simulink model "rail_ver01"  (R2018a)
settings: Solver=VariableStepAuto  StartTime=0.0  StopTime=inf  RelTol=1e-3
InitFcn:
  | %run('settingParams_ver04.m')
StopFcn:
  | run('AutomoveData.m')
values from neighbouring files (symbols this model uses):
  acceleration = 100    [settingParams_demo.m]
  armInitPos = [120,0,280,0,0,0,10,20]    [settingParams_demo.m]
  correct = [15, -50, 110, 35, 90, 90]    [settingParams_demo.m]
  direction = -1    [settingParams_demo.m]
  dt = 0.1    [settingParams_demo.m]
  dummyDepth = 600    [settingParams_demo.m]
  erosion = 1    [settingParams_demo.m]
  first = 0    [settingParams_demo.m]
  limit_range_ANA = [h2_1, h2_2, w2_r1, w2_r2, w2_l1, w2_l2]    [settingParams_demo.m]
  limit_range_IMG = [h1_1, h1_2, w1_r1, w1_r2, w1_l1, w1_l2]    [settingParams_demo.m]
  pitchAdd = [0,0,50,0,60,0]    [settingParams_demo.m]
  range_m = range / 1000    (= 0.9)    [settingParams_demo.m]
  range_mm = range    (= 900)    [settingParams_demo.m]
  relationOfArmCam = [530, 330, -100]    [settingParams_demo.m]
  termDistance = railDistance - robotLength - first    (= 0.8)    [settingParams_demo.m]
  translationVector = [0, 0, 0]    [settingParams_demo.m]
  value = [HMin, HMax, SMin, SMax, VMin, VMax]    [settingParams_demo.m]
  velocity = 50    [settingParams_demo.m]
undefined symbols (not defined in the file or in its folder): BodyIndexFrame, BodyTrackingID, ColorJointIndices, DepthJointIndices, gray, HandLeftConfidence, HandLeftState, HandRightConfidence, HandRightState, IsBodyTracked, JointPositions, JointTrackingState, none, serial, strel, videoinput
libraries: instrumentlib x6, simulink x4, visiontextngfix x3, visionmorphops x2, imaqlib x2, visionstatistics x1, sldrtlib x1
(part 1 of 2)
settings Model: Creator=tomato  LastModifiedBy=tomatoPC
settings CodeAppCC: StateflowObjectComments=on

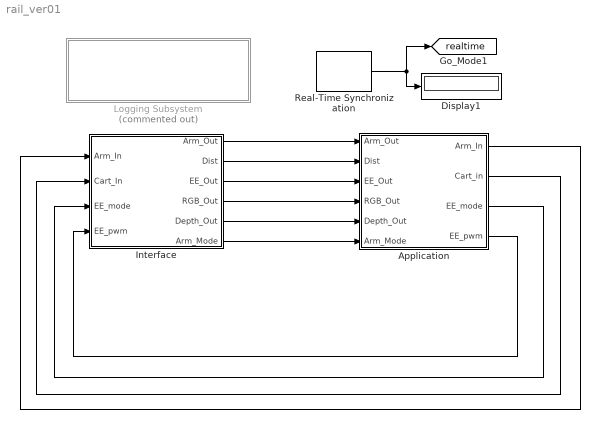
== system rail_ver01 ==
  Application : Subsystem
  Display1 : Display
  Interface : Subsystem
  Logging Subsystem : Subsystem  Commented=on
  Real-Time Synchronization : sldrtlib/Real-Time Synchronization  SampleTime=dt  MaxMissedTicks=inf  ShowMissedTicks=on  YieldWhenWaiting=off
  tag scope: realtime=global
  wires:
  Real-Time Synchronization/1 -> [realtime], Display1/1
  Application/1(Arm_In) -> Interface/1(Arm_In)
  Application/3(EE_mode) -> Interface/3(EE_mode)
  Application/2(Cart_in) -> Interface/2(Cart_In)
  Interface/1(Arm_Out) -> Application/1(Arm_Out)
  Interface/2(Dist) -> Application/2(Dist)
  Interface/3(EE_Out) -> Application/3(EE_Out)
  Interface/4(RGB_Out) -> Application/4(RGB_Out)
  Interface/5(Depth_Out) -> Application/5(Depth_Out)
  Interface/6(Arm_Mode) -> Application/6(Arm_Mode)
  Application/4(EE_pwm) -> Interface/4(EE_pwm)

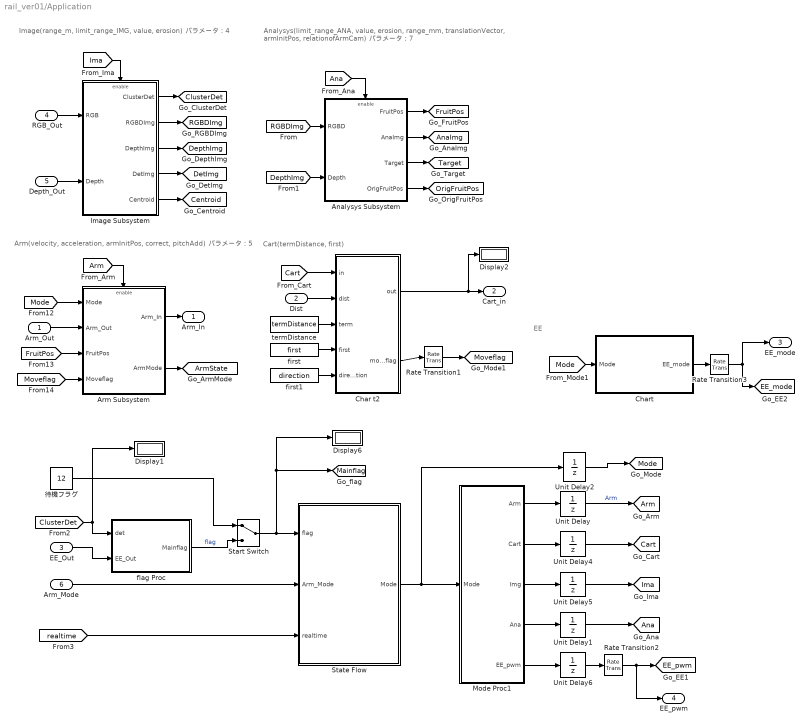
== system rail_ver01/Application ==
  note: Cart(termDistance, first)
  note: Image(range_m, limit_range_IMG, value, erosion)
      | パラメータ：4
  note: Analysys(limit_range_ANA, value, erosion, range_mm,
      |              translationVector, armInitPos, relationofArmCam)
      | パラメータ：7
  note: Arm(velocity, acceleration, armInitPos, correct, pitchAdd)
      | パラメータ：5
  note: EE
  Arm_Out : Inport
  Dist : Inport  Port=2
  EE_Out : Inport  Port=3
  RGB_Out : Inport  Port=4
  Depth_Out : Inport  Port=5
  Arm_Mode : Inport  Port=6
  Analysys Subsystem : Subsystem  TreatAsAtomicUnit=on
  Arm Subsystem : Subsystem  TreatAsAtomicUnit=on
  Char t2 : Stateflow chart  TreatAsAtomicUnit=on
  Chart : Stateflow chart  TreatAsAtomicUnit=on
  Display1 : Display
  Display2 : Display
  Display6 : Display
  Image Subsystem : Subsystem  TreatAsAtomicUnit=on
  Mode Proc1 : MATLAB Function  TreatAsAtomicUnit=on
  Rate Transition1 : RateTransition  OutPortSampleTime=0.1
  Rate Transition2 : RateTransition  OutPortSampleTime=0.1
  Rate Transition3 : RateTransition  OutPortSampleTime=0.1
  Start Switch : ManualSwitch
  State Flow : Stateflow chart  TreatAsAtomicUnit=on
  Unit Delay{,1..2,4..6} (6 alike) : UnitDelay  SampleTime=-1
  first : Constant  Value=first  SampleTime=dt
  first1 : Constant  Value=direction  SampleTime=dt
  flag Proc : MATLAB Function  TreatAsAtomicUnit=on
  termDistance : Constant  Value=termDistance  SampleTime=dt
  待機フラグ : Constant  Value=12
  Arm_In : Outport
  Cart_in : Outport  Port=2
  EE_mode : Outport  Port=3
  EE_pwm : Outport  Port=4
  tag scope: Ana=global, AnaImg=global, Arm=global, ArmState=global, Cart=global, Centroid=global, ClusterDet=global, DepthImg=global, DetImg=global, EE_mode=global, EE_pwm=global, FruitPos=global, Ima=global, Mainflag=global, Mode=global, Moveflag=global, OrigFruitPos=global, RGBDImg=global, Target=global
  wires:
  Mode Proc1/1(Arm) -> Unit Delay/1
  Mode Proc1/2(Cart) -> Unit Delay4/1
  Mode Proc1/3(Img) -> Unit Delay5/1
  Mode Proc1/5(EE_pwm) -> Unit Delay6/1
  Unit Delay/1 -> [Arm]  "Arm"
  Unit Delay5/1 -> [Ima]
  flag Proc/1(Mainflag) -> Start Switch/2  "flag"
  Start Switch/1 -> [Mainflag], Display6/1, State Flow/1(flag)
  待機フラグ/1 -> Start Switch/1
  [Arm] -> Arm Subsystem/Enable
  Arm Subsystem/1(Arm_In) -> Arm_In/1
  [FruitPos] -> Arm Subsystem/3(FruitPos)
  EE_Out/1 -> flag Proc/2(EE_Out)
  [ClusterDet] -> Display1/1, flag Proc/1(det)
  RGB_Out/1 -> Image Subsystem/1(RGB)
  Image Subsystem/1(ClusterDet) -> [ClusterDet]
  [Ima] -> Image Subsystem/Enable
  Image Subsystem/2(RGBDImg) -> [RGBDImg]
  Analysys Subsystem/1(FruitPos) -> [FruitPos]
  Mode Proc1/4(Ana) -> Unit Delay1/1
  Unit Delay1/1 -> [Ana]
  [Ana] -> Analysys Subsystem/Enable
  [RGBDImg] -> Analysys Subsystem/1(RGBD)
  Depth_Out/1 -> Image Subsystem/2(Depth)
  Arm_Mode/1 -> State Flow/2(Arm_Mode)
  State Flow/1(Mode) -> Unit Delay2/1, Mode Proc1/1(Mode)
  Unit Delay2/1 -> [Mode]
  Image Subsystem/3(DepthImg) -> [DepthImg]
  [DepthImg] -> Analysys Subsystem/2(Depth)
  Arm Subsystem/2(ArmMode) -> [ArmState]
  [Mode] -> Arm Subsystem/1(Mode)
  Arm_Out/1 -> Arm Subsystem/2(Arm_Out)
  Dist/1 -> Char t2/2(dist)
  Char t2/1(out) -> Display2/1, Cart_in/1
  termDistance/1 -> Char t2/3(term)
  first/1 -> Char t2/4(first)
  Unit Delay4/1 -> [Cart]
  [Cart] -> Char t2/1(in)
  [Moveflag] -> Arm Subsystem/4(Moveflag)
  Char t2/2(moveflag) -> Rate Transition1/1
  Image Subsystem/4(DetImg) -> [DetImg]
  Image Subsystem/5(Centroid) -> [Centroid]
  Analysys Subsystem/2(AnaImg) -> [AnaImg]
  Analysys Subsystem/3(Target) -> [Target]
  Analysys Subsystem/4(OrigFruitPos) -> [OrigFruitPos]
  [Mode] -> Chart/1(Mode)
  Chart/1(EE_mode) -> Rate Transition3/1
  Rate Transition1/1 -> [Moveflag]
  Unit Delay6/1 -> Rate Transition2/1
  Rate Transition3/1 -> [EE_mode], EE_mode/1
  Rate Transition2/1 -> EE_pwm/1, [EE_pwm]
  [realtime] -> State Flow/3(realtime)
  first1/1 -> Char t2/5(direction)

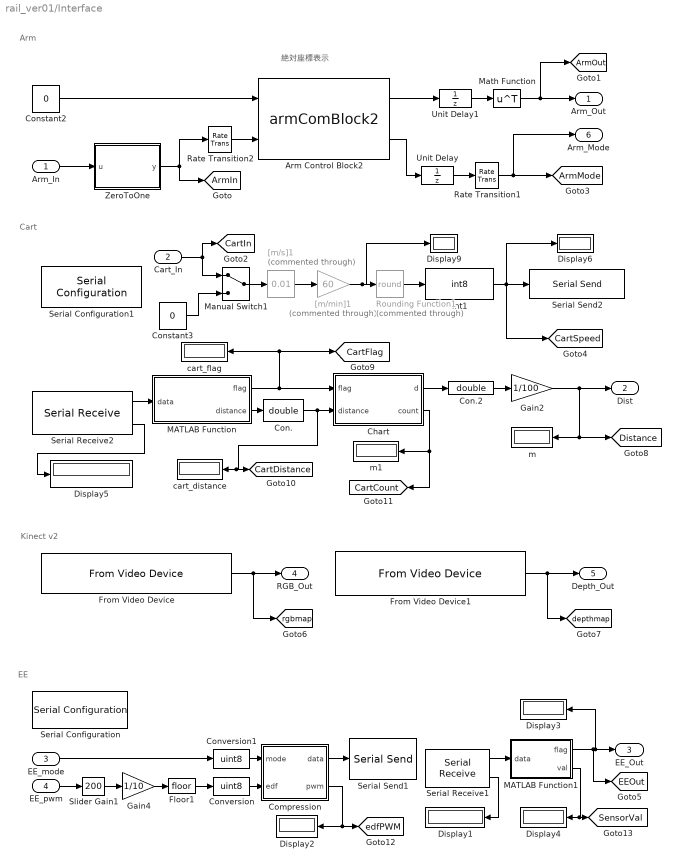
== system rail_ver01/Interface ==
  note: Kinect v2
  note: Arm
  note: 絶対座標表示
  note: EE
  note: Cart
  Arm_In : Inport
  Cart_In : Inport  Port=2
  EE_mode : Inport  Port=3
  EE_pwm : Inport  Port=4
  Arm Control Block2 : M-S-Function  FunctionName=armComBlock2  Parameters=comport, baud, tempPos  mask{comport='COM7', baud=115200, tempPos=armInitPos}
      mask prompts: comport "Port Number"; baud "Baudrate"; tempPos "Temporary Position"
      mask help: Canon Arm Control Block ver.0.8
      mask Display:
      | disp('Arm Control Block');
      | port_label('input',1,'Calib.');
      | port_label('input',2,'Target');
      | port_label('output',1,'Pos.');
      | port_label('output',2,'Moved');
  Chart : Stateflow chart  TreatAsAtomicUnit=on
  Compression : MATLAB Function  TreatAsAtomicUnit=on
  Con. : DataTypeConversion  OutDataTypeStr=double
  Con.2 : DataTypeConversion  OutDataTypeStr=double
  Constant2 : Constant  Value=0  SampleTime=0.1
  Constant3 : Constant  Value=0  SampleTime=dt
  Conversion : DataTypeConversion  OutDataTypeStr=uint8
  Conversion1 : DataTypeConversion  OutDataTypeStr=uint8
  Display{1..6,9} (7 alike) : Display
  Floor1 : Rounding
  From Video Device : imaqlib/From Video Device  DeviceMenu=kinect 1 (Kinect V2 Color Sensor)  Device=kinect 1 (Kinect V2 Color Sensor)  ObjConstructor=videoinput('kinect', 1)  VideoFormatMenu=BGR_1920x1080  VideoFormat=BGR_1920x1080  VideoSource=Kinect V2 Color Source  ROIPosition=[0 0 1080 1920]  EnableHWTrigger=off  TriggerConfiguration=kinect 1 (Kinect V2 Color Sensor)  SampleTime=0.1  OutputPortsMode=One multidimensional signal  DataType=uint8  CanDoHWTrigger=no  ReturnedColorSpace=rgb  BlockHandle=6.0001  ROIWidth=1920  ROIHeight=1080  ROIColumn=0  ROIRow=0  EngXMLPath=C:\Program Files\MATLAB\R2018a\toolbox\imaq\imaq\private  DevXMLPath=C:\ProgramData\MATLAB\SupportPackages\R2018a\toolbox\imaq\supportpackages\kinectruntime\adaptor\win64  EngLibPath=C:\Program Files\MATLAB\R2018a\toolbox\imaq\imaqblks\imaqmex\win64  ColorSpace=rgb  BayerSensorAlignment=grbg
      settings: SourceProductName=Image Acquisition Toolbox
  From Video Device1 : imaqlib/From Video Device  DeviceMenu=kinect 2 (Kinect V2 Depth Sensor)  Device=kinect 2 (Kinect V2 Depth Sensor)  ObjConstructor=videoinput('kinect', 2)  VideoFormatMenu=Depth_512x424  VideoFormat=Depth_512x424  VideoSource=Kinect V2 Depth Source  ROIPosition=[0 0 424 512]  EnableHWTrigger=off  TriggerConfiguration=none/none  SampleTime=0.1  OutputPortsMode=One multidimensional signal  DataType=uint16  CanDoHWTrigger=no  ReturnedColorSpace=grayscale  BlockHandle=6.0001  ROIWidth=512  ROIHeight=424  ROIColumn=0  ROIRow=0  EngXMLPath=C:\Program Files\MATLAB\R2018a\toolbox\imaq\imaq\private  DevXMLPath=C:\ProgramData\MATLAB\SupportPackages\R2018a\toolbox\imaq\supportpackages\kinectruntime\adaptor\win64  EngLibPath=C:\Program Files\MATLAB\R2018a\toolbox\imaq\imaqblks\imaqmex\win64  ColorSpace=grayscale  BayerSensorAlignment=grbg  AllMetadata=BodyIndexFrame;BodyTrackingID;ColorJointIndices;DepthJointIndices;HandLeftConfidence;HandLeftState;HandRightConfidence;HandRightState;IsBodyTracked;JointPositions;JointTrackingState
      settings: SourceProductName=Image Acquisition Toolbox
  Gain2 : Gain  Gain=1/100
  Gain4 : Gain  Gain=1/10
  MATLAB Function : MATLAB Function  TreatAsAtomicUnit=on
  MATLAB Function1 : MATLAB Function  TreatAsAtomicUnit=on
  Manual Switch1 : ManualSwitch
  Math Function : Math  Operator=transpose  SaturateOnIntegerOverflow=on
  Rate Transition1 : RateTransition  OutPortSampleTime=dt
  Rate Transition2 : RateTransition  OutPortSampleTime=dt
  Rounding Function1 : Rounding  Commented=through  Operator=round
  Serial Configuration : instrumentlib/Serial Configuration  Priority=-200000  ComPortMenu=<Please select a port...>  ComPort=COM3  ObjConstructor=serial('COM3');  BaudRate=115200  DataBits=8  Parity=none  StopBits=1  FlowControl=none  Timeout=10  ByteOrder=LittleEndian
  Serial Configuration1 : instrumentlib/Serial Configuration  Priority=-200000  ComPortMenu=<Please select a port...>  ComPort=COM5  ObjConstructor=serial('COM5');  BaudRate=115200  DataBits=8  Parity=none  StopBits=1  FlowControl=none  Timeout=10  ByteOrder=LittleEndian
  Serial Receive1 : instrumentlib/Serial Receive  ComPortMenu=<Please select a port...>  ComPort=COM3  ObjConstructor=serial('COM3');  Terminator=<none>  DataSize=1  DataType=uint8  EnableBlockingMode=off  ActionDataUnavailable=Output last received value  CustomValue=0  SampleTime=0.1
  Serial Receive2 : instrumentlib/Serial Receive  ComPortMenu=<Please select a port...>  ComPort=COM5  ObjConstructor=serial('COM5');  Terminator=<none>  DataSize=1  DataType=uint8  EnableBlockingMode=off  ActionDataUnavailable=Output last received value  CustomValue=0  SampleTime=0.1
  Serial Send1 : instrumentlib/Serial Send  ComPortMenu=<Please select a port...>  ComPort=COM3  ObjConstructor=serial('COM3');  Terminator=<none>  EnableBlockingMode=off
  Serial Send2 : instrumentlib/Serial Send  ComPortMenu=<Please select a port...>  ComPort=COM5  ObjConstructor=serial('COM5');  Terminator=<none>  EnableBlockingMode=on
  Slider Gain1 : simulink/Math Operations/Slider Gain  gain=200  low=0  high=250
  Unit Delay : UnitDelay  SampleTime=-1
  Unit Delay1 : UnitDelay  InitialCondition=[200 0 400 0 0 0]  SampleTime=-1
  ZeroToOne : MATLAB Function  TreatAsAtomicUnit=on
  "[m/min]1" : Gain  Commented=through  Gain=60
  "[m/s]1" : simulink/Math Operations/Slider Gain  Commented=through  gain=0.01  low=-0.23  high=0.23
  cart_distance : Display
  cart_flag : Display
  int1 : DataTypeConversion  OutDataTypeStr=int8
  m : Display
  m1 : Display
  Arm_Out : Outport
  Dist : Outport  Port=2
  EE_Out : Outport  Port=3
  RGB_Out : Outport  Port=4
  Depth_Out : Outport  Port=5
  Arm_Mode : Outport  Port=6
  tag scope: ArmIn=global, ArmMode=global, ArmOut=global, CartCount=global, CartDistance=global, CartFlag=global, CartIn=global, CartSpeed=global, Distance=global, EEOut=global, SensorVal=global, depthmap=global, edfPWM=global, rgbmap=global
  wires:
  Constant2/1 -> Arm Control Block2/1
  Arm Control Block2/1 -> Unit Delay1/1
  Math Function/1 -> [ArmOut], Arm_Out/1
  Unit Delay/1 -> Rate Transition1/1
  Arm Control Block2/2 -> Unit Delay/1
  Unit Delay1/1 -> Math Function/1
  Serial Receive1/2 -> Display1/1
  From Video Device/1 -> [rgbmap], RGB_Out/1
  From Video Device1/1 -> [depthmap], Depth_Out/1
  Manual Switch1/1 -> "[m/s]1"/1
  Cart_In/1 -> Manual Switch1/1, [CartIn]
  Rounding Function1/1 -> int1/1
  Constant3/1 -> Manual Switch1/2
  "[m/s]1"/1 -> "[m/min]1"/1
  int1/1 -> [CartSpeed], Serial Send2/1, Display6/1
  "[m/min]1"/1 -> Display9/1, Rounding Function1/1
  Serial Receive2/2 -> Display5/1
  Gain2/1 -> Dist/1, m/1, [Distance]
  Con.2/1 -> Gain2/1
  Serial Receive2/1 -> MATLAB Function/1(data)
  Chart/1(d) -> Con.2/1
  MATLAB Function/1(flag) -> cart_flag/1, [CartFlag], Chart/1(flag)
  MATLAB Function/2(distance) -> Con./1
  Chart/2(count) -> [CartCount], m1/1
  EE_pwm/1 -> Slider Gain1/1
  Gain4/1 -> Floor1/1
  Slider Gain1/1 -> Gain4/1
  Floor1/1 -> Conversion/1
  EE_mode/1 -> Conversion1/1
  Compression/1(data) -> Serial Send1/1
  Serial Receive1/1 -> MATLAB Function1/1(data)
  MATLAB Function1/2(val) -> [SensorVal], Display4/1
  Conversion/1 -> Compression/2(edf)
  Conversion1/1 -> Compression/1(mode)
  MATLAB Function1/1(flag) -> Display3/1, EE_Out/1, [EEOut]
  Con./1 -> cart_distance/1, [CartDistance], Chart/2(distance)
  Compression/2(pwm) -> [edfPWM], Display2/1
  ZeroToOne/1(y) -> Rate Transition2/1, [ArmIn]
  Rate Transition1/1 -> [ArmMode], Arm_Mode/1
  Rate Transition2/1 -> Arm Control Block2/2
  Arm_In/1 -> ZeroToOne/1(u)

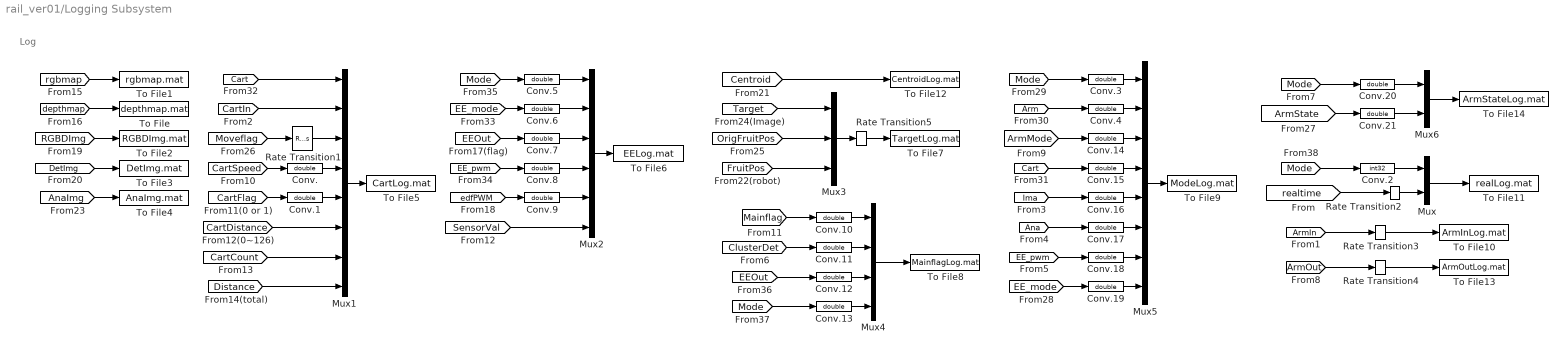
== system rail_ver01/Logging Subsystem ==
  note: Log
  Conv.{,1,3..21} (21 alike) : DataTypeConversion  OutDataTypeStr=double
  Conv.2 : DataTypeConversion  OutDataTypeStr=int32
  Mux : Mux  Inputs=2
  Mux1 : Mux  Inputs=8
  Mux2 : Mux  Inputs=6
  Mux3 : Mux  Inputs=3
  Mux4 : Mux
  Mux5 : Mux  Inputs=8
  Mux6 : Mux  Inputs=2
  Rate Transition1 : RateTransition  OutPortSampleTime=dt
  Rate Transition2 : RateTransition  OutPortSampleTime=dt
  Rate Transition3 : RateTransition  OutPortSampleTime=1
  Rate Transition4 : RateTransition  OutPortSampleTime=1
  Rate Transition5 : RateTransition  OutPortSampleTime=1
  To File : ToFile  Filename=depthmap.mat  MatrixName=depthmap  SaveFormat=Timeseries
  To File1 : ToFile  Filename=rgbmap.mat  MatrixName=rgbmap  SaveFormat=Timeseries
  To File10 : ToFile  Filename=ArmInLog.mat  MatrixName=ArmInLog  SaveFormat=Timeseries
  To File11 : ToFile  Filename=realLog.mat  MatrixName=realLog  SaveFormat=Timeseries
  To File12 : ToFile  Filename=CentroidLog.mat  MatrixName=CentroidLog  SaveFormat=Timeseries
  To File13 : ToFile  Filename=ArmOutLog.mat  MatrixName=ArmOutLog  SaveFormat=Timeseries
  To File14 : ToFile  Filename=ArmStateLog.mat  MatrixName=ArmStateLog  SaveFormat=Timeseries
  To File2 : ToFile  Filename=RGBDImg.mat  MatrixName=RGBDImg  SaveFormat=Timeseries
  To File3 : ToFile  Filename=DetImg.mat  MatrixName=DetImg  SaveFormat=Timeseries
  To File4 : ToFile  Filename=AnaImg.mat  MatrixName=AnaImg  SaveFormat=Timeseries
  To File5 : ToFile  Filename=CartLog.mat  MatrixName=CartLog  SaveFormat=Timeseries
  To File6 : ToFile  Filename=EELog.mat  MatrixName=EELog  SaveFormat=Timeseries
  To File7 : ToFile  Filename=TargetLog.mat  MatrixName=TargetLog  SaveFormat=Timeseries
  To File8 : ToFile  Filename=MainflagLog.mat  MatrixName=MainflagLog  SaveFormat=Timeseries
  To File9 : ToFile  Filename=ModeLog.mat  MatrixName=ModeLog  SaveFormat=Timeseries
  wires:
  Conv.8/1 -> Mux2/4
  [realtime] -> Rate Transition2/1
  Mux2/1 -> To File6/1
  Mux1/1 -> To File5/1
  Conv.9/1 -> Mux2/5
  [OrigFruitPos] -> Mux3/2
  [Cart] -> Mux1/1
  [CartIn] -> Mux1/2
  [CartDistance] -> Mux1/6
  Conv.1/1 -> Mux1/5
  Conv./1 -> Mux1/4
  [Distance] -> Mux1/8
  [CartCount] -> Mux1/7
  Conv.5/1 -> Mux2/1
  [Mode] -> Conv.20/1
  [EE_pwm] -> Conv.8/1
  [Moveflag] -> Rate Transition1/1
  Conv.6/1 -> Mux2/2
  Mux3/1 -> Rate Transition5/1
  [Mode] -> Conv.5/1
  [ArmState] -> Conv.21/1
  [EEOut] -> Conv.12/1
  [Ana] -> Conv.17/1
  [Mainflag] -> Conv.10/1
  [Mode] -> Conv.13/1
  [ArmIn] -> Rate Transition3/1
  [Ima] -> Conv.16/1
  [Mode] -> Conv.3/1
  [Arm] -> Conv.4/1
  [EE_pwm] -> Conv.18/1
  [EE_mode] -> Conv.19/1
  Mux5/1 -> To File9/1
  [ClusterDet] -> Conv.11/1
  Mux4/1 -> To File8/1
  [ArmOut] -> Rate Transition4/1
  Mux6/1 -> To File14/1
  [FruitPos] -> Mux3/3
  [Centroid] -> To File12/1
  [Target] -> Mux3/1
  Conv.16/1 -> Mux5/5
  Conv.18/1 -> Mux5/7
  Conv.19/1 -> Mux5/8
  Conv.15/1 -> Mux5/4
  Conv.14/1 -> Mux5/3
  Conv.4/1 -> Mux5/2
  Conv.17/1 -> Mux5/6
  Conv.3/1 -> Mux5/1
  Conv.11/1 -> Mux4/2
  Conv.10/1 -> Mux4/1
  Conv.12/1 -> Mux4/3
  Conv.13/1 -> Mux4/4
  Rate Transition1/1 -> Mux1/3
  [edfPWM] -> Conv.9/1
  [EEOut] -> Conv.7/1
  [EE_mode] -> Conv.6/1
  Conv.20/1 -> Mux6/1
  Conv.21/1 -> Mux6/2
  Conv.2/1 -> Mux/1
  [Cart] -> Conv.15/1
  [ArmMode] -> Conv.14/1
  [DetImg] -> To File3/1
  [depthmap] -> To File/1
  [rgbmap] -> To File1/1
  [RGBDImg] -> To File2/1
  Mux/1 -> To File11/1
  [Mode] -> Conv.2/1
  [AnaImg] -> To File4/1
  [CartFlag] -> Conv.1/1
  [CartSpeed] -> Conv./1
  Conv.7/1 -> Mux2/3
  Rate Transition2/1 -> Mux/2
  [SensorVal] -> Mux2/6
  Rate Transition3/1 -> To File10/1
  Rate Transition4/1 -> To File13/1
  Rate Transition5/1 -> To File7/1

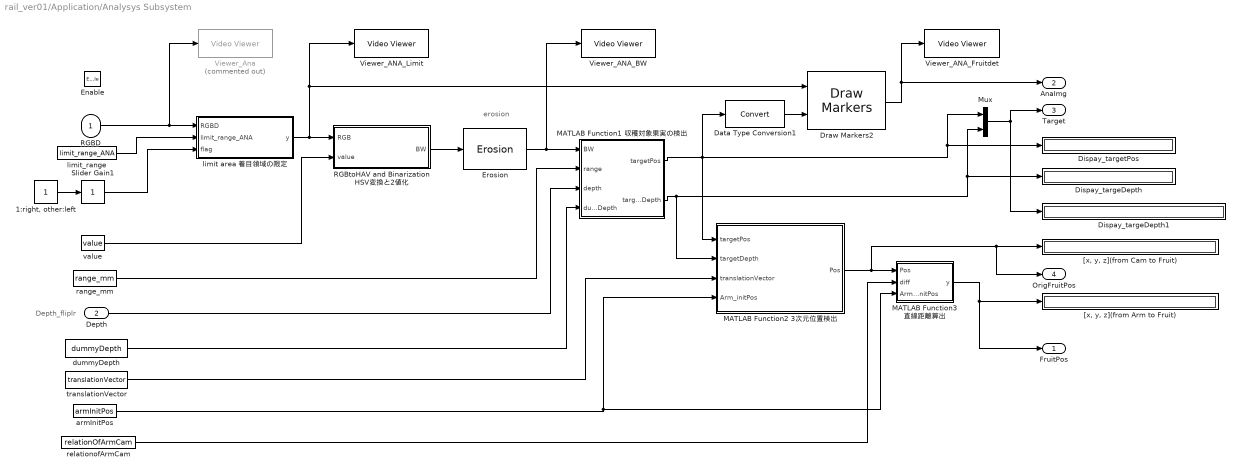
== system rail_ver01/Application/Analysys Subsystem ==
  note: Depth_fliplr
  note: erosion
  RGBD : Inport
  Depth : Inport  Port=2
  Enable : EnablePort  PropagateVarSize=During execution
  "1:right, other:left" : Constant  SampleTime=dt
  Data Type Conversion1 : DataTypeConversion
  Dispay_targeDepth : Display
  Dispay_targeDepth1 : Display
  Dispay_targetPos : Display
  Draw Markers2 : visiontextngfix/Draw Markers  shape=Circle  size=5  fill=on  fillClrSource=Specify via dialog  display=User-specified value  intensity=200  color=[0 0 255]  opacity=0.6  viewport=Entire image  antialiasing=off  inType=Obsolete  imagePorts=One multidimensional signal  prodOutputMode=Binary point scaling  prodOutputWordLength=32  prodOutputFracLength=14  memoryMode=Specify word length  memoryWordLength=16  memoryFracLength=14  roundingMode=Floor  overflowMode=off
      settings: SourceProductName=Computer Vision System Toolbox  SourceProductBaseCode=VP
  Erosion : visionmorphops/Erosion  nhoodsrc=Specify via dialog  strel=strel('disk',erosion)
      settings: SourceProductName=Computer Vision System Toolbox  SourceProductBaseCode=VP
  MATLAB Function1 収穫対象果実の検出 : MATLAB Function  TreatAsAtomicUnit=on
  MATLAB Function2 3次元位置検出 : MATLAB Function  TreatAsAtomicUnit=on
  MATLAB Function3 直線距離算出 : MATLAB Function  TreatAsAtomicUnit=on
  Mux : Mux  Inputs=2
  RGBtoHAV and Binarization HSV変換と2値化 : MATLAB Function  TreatAsAtomicUnit=on
  Slider Gain1 : simulink/Math Operations/Slider Gain  gain=1  low=0  high=2
  Viewer_ANA_BW : VideoViewer  colormapValue=gray(256)  FigPos=[1507 804 358 276]
  Viewer_ANA_Fruitdet : VideoViewer  colormapValue=gray(256)  FigPos=[1523 1037 354 274]
  Viewer_ANA_Limit : VideoViewer  colormapValue=gray(256)  FigPos=[1046 852 439 316]
  Viewer_Ana : VideoViewer  Commented=on  colormapValue=gray(256)  FigPos=[987 1052 418 304]
  "[x, y, z](from Arm to Fruit)" : Display
  "[x, y, z](from Cam to Fruit)" : Display
  armInitPos : Constant  Value=armInitPos  SampleTime=dt
  dummyDepth : Constant  Value=dummyDepth  SampleTime=dt
  limit area 着目領域の限定 : MATLAB Function  TreatAsAtomicUnit=on
  limit_range : Constant  Value=limit_range_ANA  SampleTime=dt
  range_mm : Constant  Value=range_mm  SampleTime=dt
  relationofArmCam : Constant  Value=relationOfArmCam  SampleTime=dt
  translationVector : Constant  Value=translationVector  SampleTime=dt
  value : Constant  Value=value  SampleTime=dt
  FruitPos : Outport
  AnaImg : Outport  Port=2
  Target : Outport  Port=3
  OrigFruitPos : Outport  Port=4
  wires:
  limit area 着目領域の限定/1(y) -> Draw Markers2/1, Viewer_ANA_Limit/1, RGBtoHAV and Binarization HSV変換と2値化/1(RGB)
  RGBtoHAV and Binarization HSV変換と2値化/1(BW) -> Erosion/1
  RGBD/1 -> Viewer_Ana/1, limit area 着目領域の限定/1(RGBD)
  "1:right, other:left"/1 -> Slider Gain1/1
  Depth/1 -> MATLAB Function1 収穫対象果実の検出/3(depth)
  Draw Markers2/1 -> Viewer_ANA_Fruitdet/1, AnaImg/1
  MATLAB Function1 収穫対象果実の検出/1(targetPos) -> MATLAB Function2 3次元位置検出/1(targetPos), Dispay_targetPos/1, Mux/1, Data Type Conversion1/1
  Data Type Conversion1/1 -> Draw Markers2/2
  value/1 -> RGBtoHAV and Binarization HSV変換と2値化/2(value)
  MATLAB Function1 収穫対象果実の検出/2(targetDepth) -> Dispay_targeDepth/1, Mux/2, MATLAB Function2 3次元位置検出/2(targetDepth)
  range_mm/1 -> MATLAB Function1 収穫対象果実の検出/2(range)
  Erosion/1 -> Viewer_ANA_BW/1, MATLAB Function1 収穫対象果実の検出/1(BW)
  MATLAB Function2 3次元位置検出/1(Pos) -> MATLAB Function3 直線距離算出/1(Pos), OrigFruitPos/1, "[x, y, z](from Cam to Fruit)"/1
  MATLAB Function3 直線距離算出/1(y) -> FruitPos/1, "[x, y, z](from Arm to Fruit)"/1
  limit_range/1 -> limit area 着目領域の限定/2(limit_range_ANA)
  Slider Gain1/1 -> limit area 着目領域の限定/3(flag)
  translationVector/1 -> MATLAB Function2 3次元位置検出/3(translationVector)
  relationofArmCam/1 -> MATLAB Function3 直線距離算出/2(diff)
  Mux/1 -> Target/1, Dispay_targeDepth1/1
  dummyDepth/1 -> MATLAB Function1 収穫対象果実の検出/4(dummyDepth)
  armInitPos/1 -> MATLAB Function3 直線距離算出/3(Arm_initPos), MATLAB Function2 3次元位置検出/4(Arm_initPos)

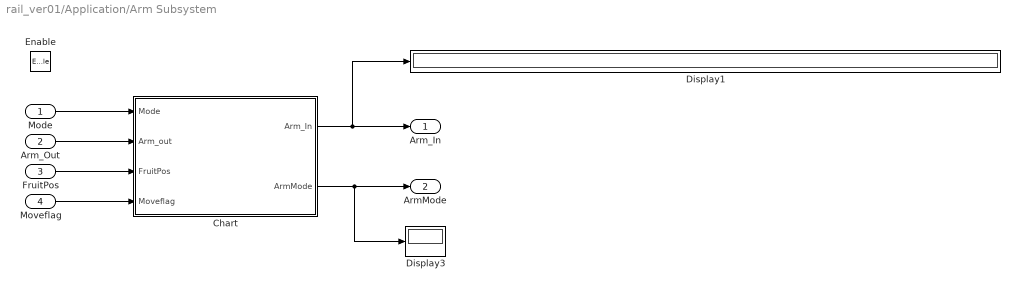
== system rail_ver01/Application/Arm Subsystem ==
  Mode : Inport  PortDimensions=1
  Arm_Out : Inport  Port=2
  FruitPos : Inport  Port=3
  Moveflag : Inport  Port=4
  Enable : EnablePort  StatesWhenEnabling=reset
  Chart : Stateflow chart  TreatAsAtomicUnit=on
  Display1 : Display
  Display3 : Display
  Arm_In : Outport  InitialOutput=armInitPos
  ArmMode : Outport  Port=2  PortDimensions=1  InitialOutput=0
  wires:
  Chart/1(Arm_In) -> Arm_In/1, Display1/1
  Arm_Out/1 -> Chart/2(Arm_out)
  Mode/1 -> Chart/1(Mode)
  Chart/2(ArmMode) -> Display3/1, ArmMode/1
  FruitPos/1 -> Chart/3(FruitPos)
  Moveflag/1 -> Chart/4(Moveflag)

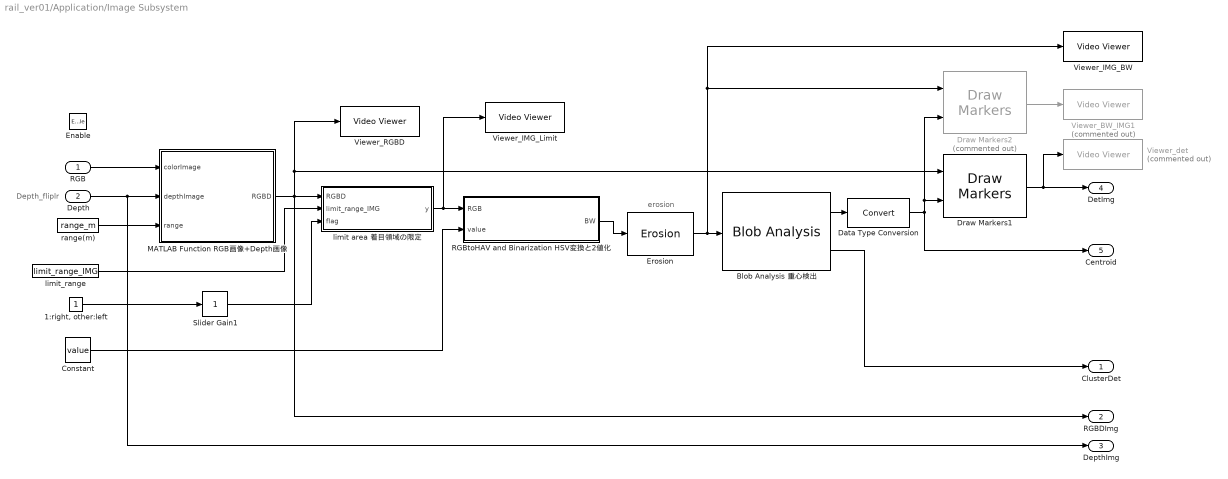
== system rail_ver01/Application/Image Subsystem ==
  note: Depth_fliplr
  note: erosion
  RGB : Inport
  Depth : Inport  Port=2
  Enable : EnablePort  StatesWhenEnabling=reset
  "1:right, other:left" : Constant  SampleTime=dt
  Blob Analysis 重心検出 : visionstatistics/Blob Analysis  Tag=vipblks_row_conv  area=off  centroid=on  bBox=off  majorAxis=off  minorAxis=off  angle=off  eccentricity=off  equivDiameterSq=off  extent=off  perimeter=off  maxBlobs=1  warnIfNumBlobsExceeded=on  isCount=on  useMinArea=off  minArea=3000  useMaxArea=off  maxArea=76800  excludeBorderBlob=off  outDT=single  isOutVarDim=off  isFill=on  fillValues=-1  conn=8  isLabel=off  outputMode=Binary point scaling  outputWordLength=32  outputFracLength=16  firstCoeffMode=Binary point scaling  firstCoeffWordLength=16  firstCoeffFracLength=14  secondCoeffMode=Binary point scaling  secondCoeffWordLength=32  secondCoeffFracLength=16  accumMode=Binary point scaling  accumWordLength=32  accumFracLength=0  prodOutputMode=Binary point scaling  prodOutputWordLength=32  prodOutputFracLength=16  roundingMode=Floor  overflowMode=off
      settings: SourceProductName=Computer Vision System Toolbox
  Constant : Constant  Value=value  SampleTime=dt
  Data Type Conversion : DataTypeConversion
  Draw Markers1 : visiontextngfix/Draw Markers  shape=Circle  size=5  fill=on  fillClrSource=Specify via dialog  display=User-specified value  intensity=200  color=[0 0 255]  opacity=0.6  viewport=Entire image  antialiasing=off  inType=Obsolete  imagePorts=One multidimensional signal  prodOutputMode=Binary point scaling  prodOutputWordLength=32  prodOutputFracLength=14  memoryMode=Specify word length  memoryWordLength=16  memoryFracLength=14  roundingMode=Floor  overflowMode=off
      settings: SourceProductName=Computer Vision System Toolbox  SourceProductBaseCode=VP
  Draw Markers2 : visiontextngfix/Draw Markers  Commented=on  shape=Star  size=1  fill=on  fillClrSource=Specify via dialog  display=Black  intensity=200  color=[0 0 255]  opacity=0.6  viewport=Entire image  antialiasing=off  inType=Obsolete  imagePorts=One multidimensional signal  prodOutputMode=Binary point scaling  prodOutputWordLength=32  prodOutputFracLength=14  memoryMode=Specify word length  memoryWordLength=16  memoryFracLength=14  roundingMode=Floor  overflowMode=off
      settings: SourceProductName=Computer Vision System Toolbox  SourceProductBaseCode=VP
  Erosion : visionmorphops/Erosion  nhoodsrc=Specify via dialog  strel=strel('disk',erosion)
      settings: SourceProductName=Computer Vision System Toolbox  SourceProductBaseCode=VP
  MATLAB Function RGB画像+Depth画像 : MATLAB Function  TreatAsAtomicUnit=on
  RGBtoHAV and Binarization HSV変換と2値化 : MATLAB Function  TreatAsAtomicUnit=on
  Slider Gain1 : simulink/Math Operations/Slider Gain  gain=1  low=0  high=2
  Viewer_BW_IMG1 : VideoViewer  Commented=on  colormapValue=gray(256)  FigPos=[1515 729 355 276]
  Viewer_IMG_BW : VideoViewer  FigPos=[1388 439 418 304]
  Viewer_IMG_Limit : VideoViewer  colormapValue=gray(256)  FigPos=[1037 437 400 321]
  Viewer_RGBD : VideoViewer  colormapValue=gray(256)  FigPos=[678 444 400 321]
  Viewer_det : VideoViewer  Commented=on  colormapValue=gray(256)  FigPos=[1453 485 453 364]
  limit area 着目領域の限定 : MATLAB Function  TreatAsAtomicUnit=on
  limit_range : Constant  Value=limit_range_IMG  SampleTime=dt
  range(m) : Constant  Value=range_m  SampleTime=dt
  ClusterDet : Outport  OutputWhenDisabled=reset  InitialOutput=0
  RGBDImg : Outport  Port=2
  DepthImg : Outport  Port=3
  DetImg : Outport  Port=4
  Centroid : Outport  Port=5
  wires:
  Depth/1 -> MATLAB Function RGB画像+Depth画像/2(depthImage), DepthImg/1
  range(m)/1 -> MATLAB Function RGB画像+Depth画像/3(range)
  RGB/1 -> MATLAB Function RGB画像+Depth画像/1(colorImage)
  Blob Analysis 重心検出/2 -> ClusterDet/1
  Draw Markers1/1 -> DetImg/1, Viewer_det/1
  Blob Analysis 重心検出/1 -> Data Type Conversion/1
  Data Type Conversion/1 -> Centroid/1, Draw Markers2/2, Draw Markers1/2
  limit_range/1 -> limit area 着目領域の限定/2(limit_range_IMG)
  MATLAB Function RGB画像+Depth画像/1(RGBD) -> RGBDImg/1, limit area 着目領域の限定/1(RGBD), Viewer_RGBD/1, Draw Markers1/1
  limit area 着目領域の限定/1(y) -> Viewer_IMG_Limit/1, RGBtoHAV and Binarization HSV変換と2値化/1(RGB)
  Constant/1 -> RGBtoHAV and Binarization HSV変換と2値化/2(value)
  Erosion/1 -> Draw Markers2/1, Viewer_IMG_BW/1, Blob Analysis 重心検出/1
  "1:right, other:left"/1 -> Slider Gain1/1
  Slider Gain1/1 -> limit area 着目領域の限定/3(flag)
  RGBtoHAV and Binarization HSV変換と2値化/1(BW) -> Erosion/1
  Draw Markers2/1 -> Viewer_BW_IMG1/1

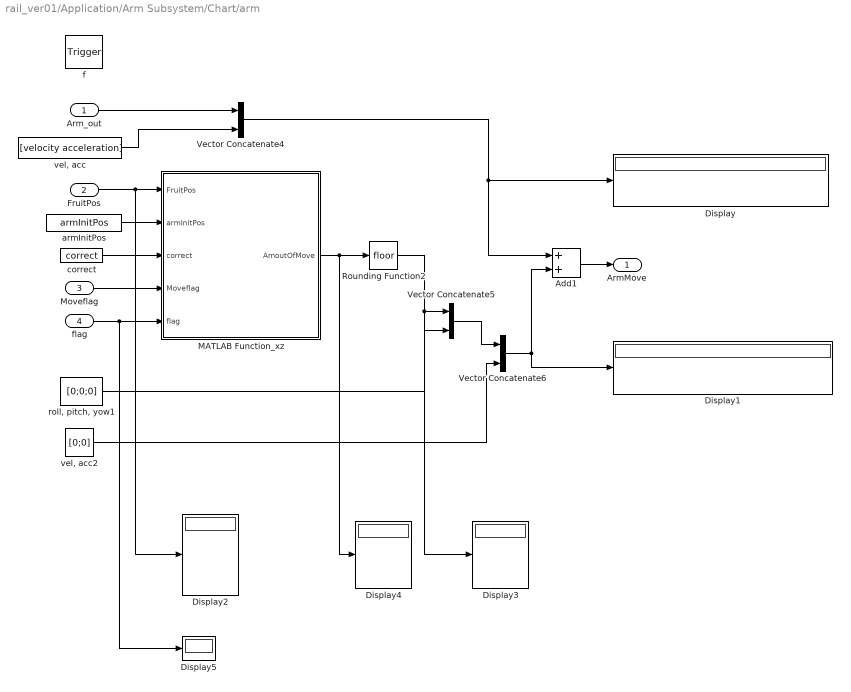
== system rail_ver01/Application/Arm Subsystem/Chart/arm ==
  Arm_out : Inport  OutDataTypeStr=double  PortDimensions=[1 6]
  FruitPos : Inport  Port=2  OutDataTypeStr=double  PortDimensions=[1 3]
  Moveflag : Inport  Port=3  OutDataTypeStr=double  PortDimensions=1
  flag : Inport  Port=4  OutDataTypeStr=double  PortDimensions=1
  f : TriggerPort  TriggerType=function-call  VariantControl=Variant
      settings: CopyFcn=Stateflow.SLINSF.SimulinkMan.removeBlockPreDeleteFcn  PreDeleteFcn=Stateflow.SLINSF.SimulinkMan.unsafePredeleteFcn
  Add1 : Sum
  Display{,1..5} (6 alike) : Display
  MATLAB Function_xz : MATLAB Function  TreatAsAtomicUnit=on
  Rounding Function2 : Rounding
  Vector Concatenate4 : Concatenate
  Vector Concatenate5 : Concatenate
  Vector Concatenate6 : Concatenate
  armInitPos : Constant  Value=armInitPos
  correct : Constant  Value=correct
  "roll, pitch, yow1" : Constant  Value=[0;0;0]
  "vel, acc" : Constant  Value=[velocity acceleration]
  "vel, acc2" : Constant  Value=[0;0]
  ArmMove : Outport  OutputWhenDisabled=reset  InitialOutput=0
  wires:
  "vel, acc"/1 -> Vector Concatenate4/2
  Arm_out/1 -> Vector Concatenate4/1
  Vector Concatenate4/1 -> Display/1, Add1/1
  "roll, pitch, yow1"/1 -> Vector Concatenate5/2
  Rounding Function2/1 -> Display3/1, Vector Concatenate5/1
  MATLAB Function_xz/1(AmoutOfMove) -> Display4/1, Rounding Function2/1
  FruitPos/1 -> Display2/1, MATLAB Function_xz/1(FruitPos)
  Vector Concatenate5/1 -> Vector Concatenate6/1
  "vel, acc2"/1 -> Vector Concatenate6/2
  Vector Concatenate6/1 -> Add1/2, Display1/1
  Add1/1 -> ArmMove/1
  Moveflag/1 -> MATLAB Function_xz/4(Moveflag)
  correct/1 -> MATLAB Function_xz/3(correct)
  armInitPos/1 -> MATLAB Function_xz/2(armInitPos)
  flag/1 -> Display5/1, MATLAB Function_xz/5(flag)

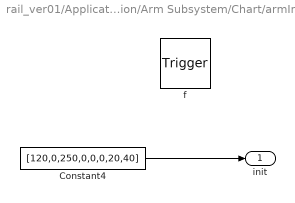
== system rail_ver01/Application/Arm Subsystem/Chart/armInit ==
  f : TriggerPort  TriggerType=function-call  VariantControl=Variant
      settings: CopyFcn=Stateflow.SLINSF.SimulinkMan.removeBlockPreDeleteFcn  PreDeleteFcn=Stateflow.SLINSF.SimulinkMan.unsafePredeleteFcn
  Constant4 : Constant  Value=[120,0,250,0,0,0,20,40]
  init : Outport  PortDimensions=[1 8]  OutputWhenDisabled=reset  InitialOutput=0
  wires:
  Constant4/1 -> init/1

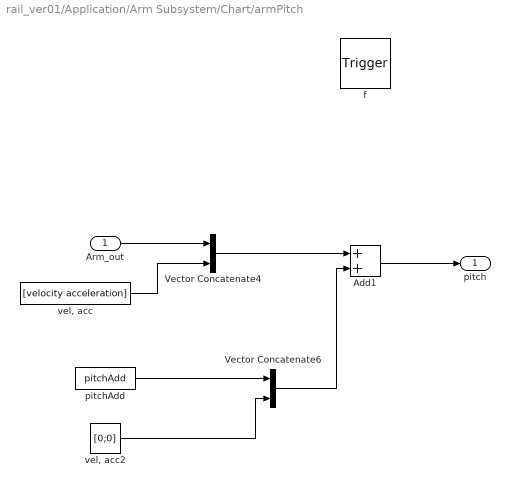
== system rail_ver01/Application/Arm Subsystem/Chart/armPitch ==
  Arm_out : Inport  OutDataTypeStr=double  PortDimensions=[1 6]
  f : TriggerPort  TriggerType=function-call  VariantControl=Variant
      settings: CopyFcn=Stateflow.SLINSF.SimulinkMan.removeBlockPreDeleteFcn  PreDeleteFcn=Stateflow.SLINSF.SimulinkMan.unsafePredeleteFcn
  Add1 : Sum
  Vector Concatenate4 : Concatenate
  Vector Concatenate6 : Concatenate
  pitchAdd : Constant  Value=pitchAdd
  "vel, acc" : Constant  Value=[velocity acceleration]
  "vel, acc2" : Constant  Value=[0;0]
  pitch : Outport  OutputWhenDisabled=reset  InitialOutput=0
  wires:
  "vel, acc"/1 -> Vector Concatenate4/2
  Arm_out/1 -> Vector Concatenate4/1
  Vector Concatenate4/1 -> Add1/1
  "vel, acc2"/1 -> Vector Concatenate6/2
  Vector Concatenate6/1 -> Add1/2
  Add1/1 -> pitch/1
  pitchAdd/1 -> Vector Concatenate6/1

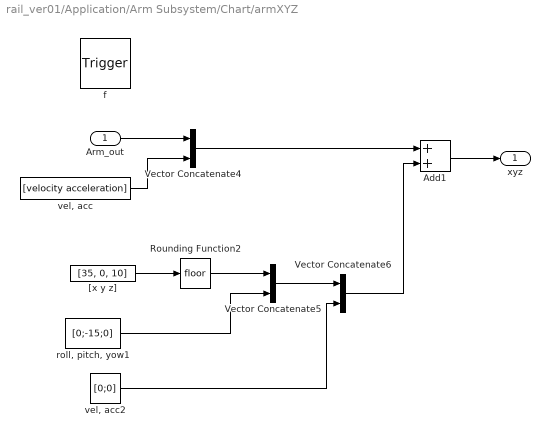
== system rail_ver01/Application/Arm Subsystem/Chart/armXYZ ==
  Arm_out : Inport  OutDataTypeStr=double  PortDimensions=[1 6]
  f : TriggerPort  TriggerType=function-call  VariantControl=Variant
      settings: CopyFcn=Stateflow.SLINSF.SimulinkMan.removeBlockPreDeleteFcn  PreDeleteFcn=Stateflow.SLINSF.SimulinkMan.unsafePredeleteFcn
  Add1 : Sum
  Rounding Function2 : Rounding
  Vector Concatenate4 : Concatenate
  Vector Concatenate5 : Concatenate
  Vector Concatenate6 : Concatenate
  "[x y z]" : Constant  Value=[35, 0, 10]
  "roll, pitch, yow1" : Constant  Value=[0;-15;0]
  "vel, acc" : Constant  Value=[velocity acceleration]
  "vel, acc2" : Constant  Value=[0;0]
  xyz : Outport  OutputWhenDisabled=reset  InitialOutput=0
  wires:
  "vel, acc"/1 -> Vector Concatenate4/2
  Arm_out/1 -> Vector Concatenate4/1
  Vector Concatenate4/1 -> Add1/1
  "roll, pitch, yow1"/1 -> Vector Concatenate5/2
  Rounding Function2/1 -> Vector Concatenate5/1
  Vector Concatenate5/1 -> Vector Concatenate6/1
  "vel, acc2"/1 -> Vector Concatenate6/2
  Vector Concatenate6/1 -> Add1/2
  Add1/1 -> xyz/1
  "[x y z]"/1 -> Rounding Function2/1

== stateflow chart rail_ver01/Application/State Flow ==
  state CheckRealtime/
    entry:Mode=-100;
  state Mode40/
    entry:Mode=40;
    % 収穫モード
    state Mode41/
      entry:Mode=41;
      % Arm(yz)移動_Arm
    state Mode42/
      entry:Mode=42;
      % Arm(x)移動・吸引_Arm, EE
    state wait40/
      entry:Mode=-40;
    state Mode43/
      entry:Mode=43;
      % 切断1(閉)_EE
    state Mode47/
      entry:
      Mode=47;
      failed=0;
      % 収穫失敗
      % 吸引なし
    state Mode46/
      entry:
      Mode=46;
      failed = 1;
      % Arm(xyz)移動
      %吸引_Arm, EE
    state Mode44/
      entry:Mode=44;
      % 切断2(開)_EE
    state Mode45/
      entry:Mode=45;
      % 把持_EE
    (default) -> Mode41
    Mode41 -> Mode42 : after(1,sec)
        | [Arm_Mode == 1]
    Mode42 -> wait40 : after(1,sec)
        | [Arm_Mode == 1]
    Mode46 -> wait40 : after(1,sec)
        | [Arm_Mode == 1]
    wait40 -> Mode43 [order 1] : [Arm_Mode == 1 && flag == 43]
        | % flag==43 : 光センサ反応
    wait40 -> Mode47 [order 2] : after(3.5,sec)
        | [failed == 1]
    wait40 -> Mode46 [order 3] : after(3.5,sec)
    Mode43 -> Mode44 : % 上SW反応
        | after(0.5,sec)
        | [flag == 44 || after(20,sec)]
    Mode45 -> Mode47 [order 2] : % 把持失敗
        | after(2,sec)
        | [flag == 46]
    Mode44 -> Mode45 : % 下SW反応
        | [after(0.5,sec)]
  state Mode10/
    entry:Mode=10;
    % 動作準備モード
    state Mode10/
      entry:Mode=11;
      % Armキャリブレーション_Arm
    state Mode12/
      entry:Mode=12;
      % 待機
    (default) -> Mode10.Mode10
    Mode10.Mode10 -> Mode12 : [Arm_Mode == 1]
    Mode12 -> Mode12 [order 1] : [flag == 12]
  state Mode20/
    entry:Mode=20;
    % 探索モード
    state Mode21/
      entry:Mode=21;
      % 微小移動_Cart
    state Mode22/
      entry:Mode=22;
      % トマト探索_Cart, Img
    (default) -> Mode21
    Mode21 -> Mode22 : %after(0,sec)
  state Mode60/
    entry:Mode=60;
    % 果実誘導モード
    state o/
      entry:Mode = 60;
    state Mode61/
      entry:Mode=61;
      % Arm(pitch)移動_Arm
    state Mode63/
      entry:Mode=62;
      %
    state Mode62/
      entry:
      Mode=62;
      count=0;
      % Arm初期位置へ移動
    (default) -> o
    o -> Mode61 : after(9,sec)
    Mode61 -> Mode63 : after(1,sec)
        | [Arm_Mode == 1]
    Mode63 -> Mode62 : [after(2,sec)]
  state Mode50/
    entry:Mode=50;
    % 完了モード
    state Mode51/
      entry:Mode=51;
      % Arm初期位置へ_Arm
    state wait50/
      entry:Mode=-50;
    (default) -> Mode51
    Mode51 -> wait50 : after(1,sec)
        | [Arm_Mode == 1]
  state Mode30/
    entry:Mode=30;
    % 解析モード
    state Mode31/
      entry:Mode=31;
      % 目標トマト果実位置の検出_Ana
    (default) -> Mode31
  state Mod70/
    entry:
    Mode=70;
    failed=0;
    % 終了モード
  (default) -> CheckRealtime
  CheckRealtime -> CheckRealtime [order 2]
  Mode22 -> CheckRealtime [order 2] : [realtime >1000]
  CheckRealtime -> Mode10 [order 1] : [realtime < 1000]
      | {count=0;
      | failed=0;}
  Mode12 -> Mode20 [order 2] : after(2.0,sec)
  Mode47 -> Mode50 : after(1,sec)
  Mode31 -> Mode40 : after(1,sec)
  Mode45 -> Mode50 [order 1] : % 把持成功
      | after(1,sec)
      | [flag == 50]
  Mod70 -> Mode20 : after(2,sec)
  Mode22 -> Mode30 [order 1] : [flag == 30]
  wait50 -> Mode60 [order 1] : [flag == 50]
      | % 光センサ反応
  wait50 -> Mod70 [order 2] : after(1,sec)
  Mode62 -> Mod70 : after(1,sec)
      | [Arm_Mode == 1]
  data: Mode output; flag input; Arm_Mode input; count local; failed local; realtime input

== matlab function rail_ver01/Application/Arm Subsystem/Chart/arm/MATLAB Function_xz ==
  data: FruitPos input; AmoutOfMove output; armInitPos input; correct input; Moveflag input; flag input
function AmoutOfMove = fcn(FruitPos, armInitPos, correct, Moveflag, flag)
AmoutOfMove=[0, 0, 0];
% [x, y, z](ロボット座標)

if FruitPos(1) == 0 && FruitPos(2) == 0 && FruitPos(3) == 0
    AmoutOfMove(1) = armInitPos(1);
    AmoutOfMove(2) = armInitPos(2);
    AmoutOfMove(3) = armInitPos(3);
else
    % Moveflag == 1 : 右方向
    if Moveflag == 1
        % x
        AmoutOfMove(1) = FruitPos(1) + correct(1);
        % y
        AmoutOfMove(2) = FruitPos(2) + correct(2);
        % z
        AmoutOfMove(3) = FruitPos(3) + (FruitPos(3)-100) * -0.08 + correct(3);
        
    % Moveflag == -1 : 左方向
    else
        % x
        AmoutOfMove(1) = FruitPos(1) + correct(4);
        % y
        AmoutOfMove(2) = FruitPos(2) + correct(5);
        % z
        AmoutOfMove(3) = FruitPos(3) + (FruitPos(3)-100) * -0.08 + correct(6);
    end
end

% flag == 1 : yz移動
if flag == 1
    % x方向移動量：0
    AmoutOfMove(1) = 0;

% flag == 2 : x移動
elseif flag == 2
    % yz方向移動量：0
    AmoutOfMove(2) = 0;
    AmoutOfMove(3) = 0;
else
    AmoutOfMove(1) = 0;
    AmoutOfMove(2) = 0;
    AmoutOfMove(3) = 0;
end

== stateflow chart rail_ver01/Interface/Chart ==
  state mode0/
  state mode1/
    entry:
    count = count;
    d = (count * 127) + distance;
    during:
    d = distance + count * 127;
    count = count;
  (default) -> mode0 : {
      | d = 0;
      | count = 0;
      | }
  mode0 -> mode1
  mode1 -> mode1 : [flag == 1]
      | {
      | count = count + 1;
      | }
  data: flag input; distance input; d output double; count output

== matlab function rail_ver01/Application/Analysys Subsystem/MATLAB Function1 収穫対象果実の検出 ==
  data: BW input; range input; targetPos output; depth input; targetDepth output; dummyDepth input
function [targetPos,targetDepth] = fcn(BW,range, depth, dummyDepth)
targetPos = [0, 0];
depth = fliplr(depth);
targetDepth = 0;
% %% 非ゼロ検出
[row,col] = find(BW);
 s=size(row);
 n=s(1);
 if n ~= 0
    position=zeros(n,3);
    for i=1:n
        position(i,1)=col(i);
        position(i,2)=row(i);
        position(i,3)=depth(row(i), col(i));
    end
%%
    [row2,col2, v] = find(position(:,3));

    [M, Index]=min(v);

    a=0;b=0;
    a=position(row2(Index),1);
    b=position(row2(Index),2);

    disp(position(row2(Index),1))
%%
    Dav = uint16(0);
    count = 0;
    for i = -1: 1
        for j = -1: 1
            if (BW(b + j, a + i) == 1) && (depth(b + j, a + i) ~= 0) && (depth(b + j, a + i) <= range)
                Dav = Dav + depth(b + j, a + i);
                count = count + 1;
                disp(depth(b + j, a + i));
            end
        end
    end
    Dav = Dav / count;

    if Dav == 0
        Dav = uint16(dummyDepth);
    end

    targetPos = [a, b];
    targetDepth = double(Dav);
 end

== matlab function rail_ver01/Application/Mode Proc1 ==
  data: Mode input; Arm output; Cart output; Img output; Ana output; EE_pwm output
function [Arm, Cart, Img, Ana, EE_pwm] = fcn(Mode)

Arm = 0;
Cart = 0;
Img = 0;
Ana = 0;
EE_pwm = 0;

% Cart
if Mode==21
    % 微小移動_Cart
    Cart = 1;
    
% Cart, Img
elseif Mode==22
    % トマト探索_Cart, Img
    Cart = 1;
    Img = 1;

% Ana
elseif Mode==30 || Mode==31
    % 解析モード
    % 目標トマト果実位置の検出_Ana
    Ana = 1;
% Arm
elseif Mode==41 || Mode == 61 || Mode == 62
    %Mode == 41 Arm(yz)移動_Arm
    %Mode == 61 Arm(pitch)移動_Arm
    %Mode == 62 Arm初期値へ_Arm
    Arm = 1;

% Arm, EE
elseif Mode == 42 || Mode == 46
    % Mode == 42 Arm_x, EE
    % Mode == 46 Arm_xyz, EE
    Arm = 1;
    EE_pwm = 1;
    
% EE
elseif Mode == 43 || Mode == 44  || Mode == 45 || Mode == 47 || Mode == -40 || Mode == 50 || Mode == -50 || Mode == 60 || Mode == 61
    % Mode == 43(切断1), 44(切断2), 45(把持), 47(失敗), -40
    % Mode == -50, 50
    % Mode == 60
    EE_pwm = 1;
    
% EE_EFDストップ
elseif Mode == 47
    % Mode == 47
    EE_pwm = 0;
    
% Arm, EE
elseif Mode == 50 || Mode == 51
    % Mode == 50, 51
    Arm = 1;
    EE_pwm = 1;
    
% No
else
    Arm = 0;
    Cart = 0;
    Img = 0;
    EE_pwm = 0;
    Ana = 0;
end

== matlab function rail_ver01/Application/Image Subsystem/limit area 着目領域の限定 ==
  data: RGBD input; y output; limit_range_IMG input; flag input
function y = fcn(RGBD, limit_range_IMG, flag)

% 上側除去
for i=1:limit_range_IMG(1)
    RGBD(i,:,:)=0;
end
% 下側除去
for i=limit_range_IMG(2):424
    RGBD(i,:,:)=0;
end

% 424*512pixel
% 横半分256の半分128±50pixel
% 右側着目：flag = 1 : 左側領域除去：i=78:178
% 左側着目：other    : 右側領域除去：i=334:438
    
if flag==1
    % 左側除去
    for i=1:limit_range_IMG(3)
        RGBD(:,i,:)=0;
    end
    for i=limit_range_IMG(4):512
        RGBD(:,i,:)=0;
    end
else
    % 右側除去
    for i=1:limit_range_IMG(5)
        RGBD(:,i,:)=0;
    end
    for i=limit_range_IMG(6):512
        RGBD(:,i,:)=0;
    end
end

y=RGBD;

== matlab function rail_ver01/Interface/MATLAB Function ==
  data: flag output; data input; distance output
function [flag,distance] = fcn(data)

% 入力(data)を右に7bitシフトして、上位1bitを取り出す
flag = uint8(bitshift(data,-7));

% 入力(data)と127(01111111)のAND演算をして、下位7bitを取り出す
distance = uint8( bitand(data, 127));

== matlab function rail_ver01/Application/flag Proc ==
  data: det input; Mainflag output; EE_Out input
function Mainflag = fcn(det, EE_Out)

% トマト果実検出
if det== 1
    Mainflag = 30;
% センサ反応
elseif EE_Out == 5
    Mainflag = 43;
% 上SW反応
elseif EE_Out == 6
    Mainflag = 44;
% 下SW反応
elseif EE_Out == 7
    Mainflag = 45;
% 把持中
elseif EE_Out == 4
    Mainflag = 50;
% 把持失敗
elseif EE_Out == 0
    Mainflag = 46;
else
    Mainflag = -1;
end

== matlab function rail_ver01/Application/Analysys Subsystem/MATLAB Function2 3次元位置検出 ==
  data: targetPos input; Pos output; targetDepth input; translationVector input; Arm_initPos input
function Pos = fcn(targetPos, targetDepth, translationVector ,Arm_initPos)

Pos = [targetPos(1), targetPos(2), -1];
%Depthmap=fliplr(Depthmap);

coder.extrinsic('evalin', 'pointsToWorld')
Params = evalin('base', 'IRcameraParams');
R = evalin('base', 'R');
% t = evalin('base', 't');

if targetPos(2)~=-1 && targetDepth ~= 0
    %ArmX=double(Depthmap(round(u(2)), round(u(1))));
    ArmX=double(targetDepth);
    translationVector(3)=ArmX;
    imagePoints=[targetPos(1), targetPos(2)];

    % 画像座標を世界座標へ
    worldPoints1 = pointsToWorld(Params, R, translationVector, imagePoints);
    % disp(worldPoints1(1));
    % disp(worldPoints1(2));
    ArmY=worldPoints1(1);
    ArmZ=worldPoints1(2);
    %test = round(ArmY) - 80; 
    
    Pos = [ArmX, ArmY, ArmZ];
    Pos(3) = -1 * ArmZ;     % -1をかける
    Pos(2) = Pos(2) -80;    % kinectのずれ補正
else
    Pos = [Arm_initPos(1),Arm_initPos(2), Arm_initPos(3)];
end

== stateflow chart rail_ver01/Application/Chart ==
  state m03/
    % 切断2_逆転中
    entry:
    EE_mode=3;
  state m0/
    % 待機中
    entry:
    EE_mode=0;
  state m01/
    % 吸引中
    entry:
    EE_mode=1;
  state m04/
    % 把持中
    entry:
    EE_mode=4;
  state m02/
    % 切断1_正転中
    entry:
    EE_mode=2;
  m03 -> m0 : [Mode==47 || Mode==62 || Mode==70]
  (default) -> m0
  m04 -> m0 [order 1] : [Mode==47 || Mode==62 || Mode==70]
  m02 -> m0 [order 2] : [Mode==47 || Mode==62 || Mode==70]
  m04 -> m03 [order 2] : % 下SW反応
      | [Mode == 60]
  m01 -> m0 [order 2] : % 失敗
      | [Mode == 47]
  m0 -> m01 : % 吸引開始
      | [Mode == 42]
  m02 -> m04 [order 1] : % 上SW反応
      | [Mode == 44]
  m01 -> m02 [order 1] : % 光センサ反応
      | [Mode == 43]
  data: Mode input; EE_mode output

== matlab function rail_ver01/Application/Image Subsystem/MATLAB Function RGB画像+Depth画像 ==
  data: colorImage input; RGBD output uint8 size=[424 512 3]; depthImage input; range input
function RGBD  = fcn(colorImage, depthImage, range)

coder.extrinsic('pcfromkinect')
coder.extrinsic('evalin')
coder.extrinsic('getfield')

% depthDevice = imaq.VideoDevice('kinect',2);
device = evalin('base', 'depthDevice');

pc = pcfromkinect(device,depthImage,colorImage, 'depthCentric');
a = single(zeros(424, 512,3));
b = uint8(zeros(424, 512,3));
a = getfield(pc, 'Location');
b = getfield(pc, 'Color');

for i=1:424
   for j=1:512
       if a(i,j,3) < range
           b(i,j,:)=b(i,j,:);
       else
           b(i,j,:)=255;
       end
   end
end

RGBD=b;

% y = single(zeros(424, 512));
% y = fliplr(getfield(pc, 'Location'));
% y = fliplr(y);

== matlab function rail_ver01/Application/Image Subsystem/RGBtoHAV and Binarization HSV変換と2値化 ==
  data: RGB input; BW output; value input
function BW = createMask(RGB, value)
%createMask  Threshold RGB image using auto-generated code from colorThresholder app.
%  [BW,MASKEDRGBIMAGE] = createMask(RGB) thresholds image RGB using
%  auto-generated code from the colorThresholder App. The colorspace and
%  minimum/maximum values for each channel of the colorspace were set in the
%  App and result in a binary mask BW and a composite image maskedRGBImage,
%  which shows the original RGB image values under the mask BW.

% Auto-generated by colorThresholder app on 12-Apr-2017
%------------------------------------------------------


% Convert RGB image to chosen color space
I = rgb2hsv(RGB);
%%
% H
channel1Min = value(1);
channel1Max = value(2);
% S
channel2Min = value(3);
channel2Max = value(4);
% V
channel3Min = value(5);
channel3Max = value(6);

% Create mask based on chosen histogram thresholds
sliderBW = ( (I(:,:,1) >= channel1Min) | (I(:,:,1) <= channel1Max) ) & ...
    (I(:,:,2) >= channel2Min ) & (I(:,:,2) <= channel2Max) & ...
    (I(:,:,3) >= channel3Min ) & (I(:,:,3) <= channel3Max);
%%
BW = sliderBW;

end

== matlab function rail_ver01/Application/Analysys Subsystem/limit area 着目領域の限定 ==
  data: RGBD input; y output; limit_range_ANA input; flag input
function y = fcn(RGBD, limit_range_ANA, flag)

% 上側除去
for i=1:limit_range_ANA(1)
    RGBD(i,:,:)=0;
end
% 下側除去
for i=limit_range_ANA(2):424
    RGBD(i,:,:)=0;
end

% 424*512pixel
% 横半分256の半分128±50pixel
% 右側着目：flag = 1 : 左側領域除去：i=78:178
% 左側着目：other    : 右側領域除去：i=334:438
    
if flag==1
    % 左側除去
    for i=1:limit_range_ANA(3)
        RGBD(:,i,:)=0;
    end
    for i=limit_range_ANA(4):512
        RGBD(:,i,:)=0;
    end
else
    % 右側除去
    for i=1:limit_range_ANA(5)
        RGBD(:,i,:)=0;
    end
    for i=limit_range_ANA(6):512
        RGBD(:,i,:)=0;
    end
end

y=RGBD;

== matlab function rail_ver01/Interface/ZeroToOne ==
  data: u input; y output
function y = fcn(u)
if u(7) == 0
    u(7) = 50;
end
if u(8) == 0
    u(8) = 100;
end
y = u;

== stateflow chart rail_ver01/Application/Arm Subsystem/Chart ==
  state ArmSub40/
  state ArmSub41/
    % Arm(yz)移動
    entry:
    flag=1;
    Arm_In=arm(Arm_out, FruitPos, Moveflag, flag);
    ArmMode=41;
    during:
    ArmMode=-41;
  state ArmSub44/
    % Arm(xyz)移動
    entry:
    Arm_In=armXYZ(Arm_out);
    ArmMode=44;
    during:
    ArmMode=-44;
  state ArmSub99/
    entry:
    Arm_In=armInit;
    ArmMode=99;
    during:
    ArmMode=-99;
  state ArmSub61/
    % Arm(pitch)移動
    entry:
    Arm_In=armPitch(Arm_out);
    ArmMode=61;
    during:
    ArmMode=-61;
  state ArmMove = arm(Arm_out,FruitPos,Moveflag,flag) [function]
  state xyz = armXYZ(Arm_out) [function]
  state ArmSub42/
    % Arm(x)移動
    entry:
    flag=2;
    Arm_In=arm(Arm_out, FruitPos, Moveflag, flag);
    ArmMode=42;
    during:
    ArmMode=-42;
  state pitch = armPitch(Arm_out) [function]
  state init = armInit [function]
  state ArmSub100/
    entry:ArmMode=100;
  (default) -> ArmSub40 : {
      | ArmMode=0;
      | flag=0;
      | }
  ArmSub40 -> ArmSub99 [order 4] : [Mode==51 || Mode==62]
  ArmSub100 -> ArmSub40
  ArmSub40 -> ArmSub61 [order 3] : [Mode == 61]
  ArmSub40 -> ArmSub41 [order 1] : [Mode == 41]
  ArmSub40 -> ArmSub44 [order 2] : [Mode == 46]
  ArmSub61 -> ArmSub100 : after(0.5,sec)
  ArmSub99 -> ArmSub100 : after(0.5,sec)
  ArmSub44 -> ArmSub100 : after(0.5,sec)
  ArmSub41 -> ArmSub42 : [Mode == 42]
  ArmSub42 -> ArmSub100 : after(0.5,sec)
  data: Arm_out function_input double size=[1 6]; FruitPos function_input double size=[1 3]; ArmMove function_output; Moveflag function_input double size=1; flag function_input double size=1; Arm_out function_input double size=[1 6]; xyz function_output; Arm_out function_input double size=[1 6]; pitch function_output; init function_output size=[1 8]; Mode input; Arm_out input; FruitPos input; Arm_In output size=[1 8]; ArmMode output; Moveflag input; flag local

== matlab function rail_ver01/Interface/Compression ==
  data: mode input; edf input; data output; pwm output
function [data,pwm] = fcn(mode, edf)

if mode < 0
    mode = uint8(0);
elseif mode > 7
    mode = uint8(7);
end

if edf > 25
    edf = uint8(25);
end

pwm = uint8(edf);

data = bitshift(mode,5) + pwm;

== stateflow chart rail_ver01/Application/Char t2 ==
  state CartWait/
    entry:out=0;
  state CartGo1/
    entry:out=0;
  state CartGo3/
    entry:
    flag=flag*-1;
    moveflag = flag;
    t=t+term;
  state CartGo2/
    entry:out=flag;
  (default) -> CartWait : {
      | out = 0;
      | flag=direction;
      | moveflag = flag;
      | t=term+first;
      | }
  CartGo2 -> CartWait [order 1] : [in == 0]
  CartWait -> CartGo1 : [in == 1]
  CartGo1 -> CartGo3 [order 2] : [dist >= t && abs(dist - t) <= 1 ]
  CartGo1 -> CartGo2 [order 1] : [dist < t ]
  CartGo2 -> CartGo3 [order 2] : [dist >= t && abs(dist - t) <= 1]
  CartGo3 -> CartGo2
  data: in input; out output; dist input; term input; flag local; t local; first input double size=1; moveflag output; direction input

== matlab function rail_ver01/Interface/MATLAB Function1 ==
  data: flag output; data input; val output
function [flag,val] = fcn(data)

% 入力(data)を右に5bitシフトして、上位3bitを取り出す
flag = uint8(bitshift(data,-5));

% 入力(data)と31(00011111)のAND演算をして、下位5bitを取り出す
a = double( bitand(data, 31));

val = a * 10 + 800;

== matlab function rail_ver01/Application/Analysys Subsystem/MATLAB Function3 直線距離算出 ==
  data: Pos input; y output; diff input; Arm_initPos input
function y = fcn(Pos, diff, Arm_initPos)
y=[0, 0, 0];
% [x, y, z](Arm座標)
% x
if Pos(1) == Arm_initPos(1)
    y(1) = 0;
    y(2) = 0;
    y(3) = 0;
else
    % 直線距離の算出
    Pos(1)=Pos(1)*cos(asin((Pos(2))/Pos(1)));
    y(1) = Pos(1)-diff(1); 
    % y
    y(2) = diff(2)-Pos(2);
    % z
    %y(3) = diff(3)-pos(3);
    y(3) = Pos(3) - diff(3);
end
